simulink library "threeSurfaceThreeTether_cl"  (R2018b)
settings: Solver=VariableStepAuto  StartTime=0.0  StopTime=10.0  RelTol=1e-3
libraries: vrlib x4, aeroSurface_ul x4, apparentWind_ul x1, eulAng2RotMat_ul x1, vectorNormalizer_ul x1, sixDoFKinematics_ul x1
settings Model: Creator=mcobb  LastModifiedBy=mcobb

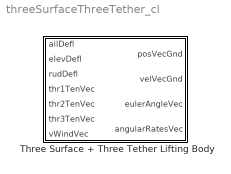
== system threeSurfaceThreeTether_cl ==
  Three Surface + Three Tether Lifting Body : Subsystem  mask{rho=1.225, vol=1, grav=9.81, thr1PosVec=[1 0 0], thr2PosVec=[1 0 0], thr3PosVec=[1 0 0], CB2CMVec=[1 0 0], m=1, inertiaMatrix=eye(3), initPos=[0 0 0], initVel=[0 0 0], initEulerAngles=[0 0 0], initAngRates=[0 0 0], hStabWingAeroCentVec=[0 0 0], hStabRotVec=[1 0 0], hStabChordVec=[0 1 0], hStabRefArea=1, hStabLiftCoeffFitParams=[1 0], hStabDragCoeffFitParams=[1 0 0], vStabWingAeroCentVec=[0 0 0], vStabRotVec=[1 0 0], vStabChordVec=[0 1 0], vStabRefArea=1, vStabLiftCoeffFitParams=[1 0], vStabDragCoeffFitParams=[1 0 0], prtWingAeroCentVec=[0 0 0], prtRotVec=[1 0 0], prtChordVec=[0 1 0], prtRefArea=1, prtLiftCoeffFitParams=[1 0], prtDragCoeffFitParams=[1 0 0], sbdWingAeroCentVec=[0 0 0], sbdRotVec=[1 0 0], sbdChordVec=[0 1 0], sbdRefArea=1, sbdLiftCoeffFitParams=[1 0], sbdDragCoeffFitParams=[1 0 0]}
      mask prompts: rho "Fuild Density"; vol "Volume"; grav "Gravity"; thr1PosVec "Tether 1"; thr2PosVec "Tether 2"; thr3PosVec "Tether 3"; CB2CMVec "CoM 2 CoB Vec"; m "Mass"; inertiaMatrix "Inertia matrix"; initPos "Initial position vec"; initVel "Initial velocity vec"; initEulerAngles "Initial euler angles"; initAngRates "Initial angular rates vec"; hStabWingAeroCentVec "Aerodynamic Center Vec"; hStabRotVec "Spanwise Rotation Vector"; hStabChordVec "Chord Direction Vec"; hStabRefArea "Ref Area"; hStabLiftCoeffFitParams "Lift Coefficient Fit Parameters"; hStabDragCoeffFitParams "Drag Coefficient Fit Parameters"; vStabWingAeroCentVec "Aerodynamic Center Vec"; vStabRotVec "Spanwise Rotation Vector"; vStabChordVec "Chord Direction Vec"; vStabRefArea "Ref Area"; vStabLiftCoeffFitParams "Lift Coefficient Fit Parameters"; vStabDragCoeffFitParams "Drag Coefficient Fit Parameters"; prtWingAeroCentVec "Aerodynamic Center Vec"; prtRotVec "Spanwise Rotation Vector"; prtChordVec "Chord Direction Vec"; prtRefArea "Ref Area"; prtLiftCoeffFitParams "Lift Coefficient Fit Parameters"; prtDragCoeffFitParams "Drag Coefficient Fit Parameters"; sbdWingAeroCentVec "Aerodynamic Center Vec"; sbdRotVec "Spanwise Rotation Vector"; sbdChordVec "Chord Direction Vec"; sbdRefArea "Ref Area"; sbdLiftCoeffFitParams "Lift Coefficient Fit Parameters"; sbdDragCoeffFitParams "Drag Coefficient Fit Parameters"
      mask DialogControl Container8 Prompt: Parameters
      mask DialogControl ParameterGroupVar Prompt: Environmental
      mask DialogControl Container3 Prompt: Tether attachment positiong vecs in body frame
      mask DialogControl Container4 Prompt: Cent of mass 2 cent of buoy vec
      mask DialogControl Container5 Prompt: Inertial Settings
      mask DialogControl Container11 Prompt: Horz. Stab.
      mask DialogControl Container14 Prompt: Aerodynamic Parameters
      mask DialogControl Container16 Prompt: Vert. Stab.
      mask DialogControl Container15 Prompt: Aerodynamic Parameters
      mask DialogControl Container17 Prompt: Port Wing
      mask DialogControl Container12 Prompt: Aerodynamic Parameters
      mask DialogControl Container18 Prompt: Stb. Wing
      mask DialogControl Container13 Prompt: Aerodynamic Parameters

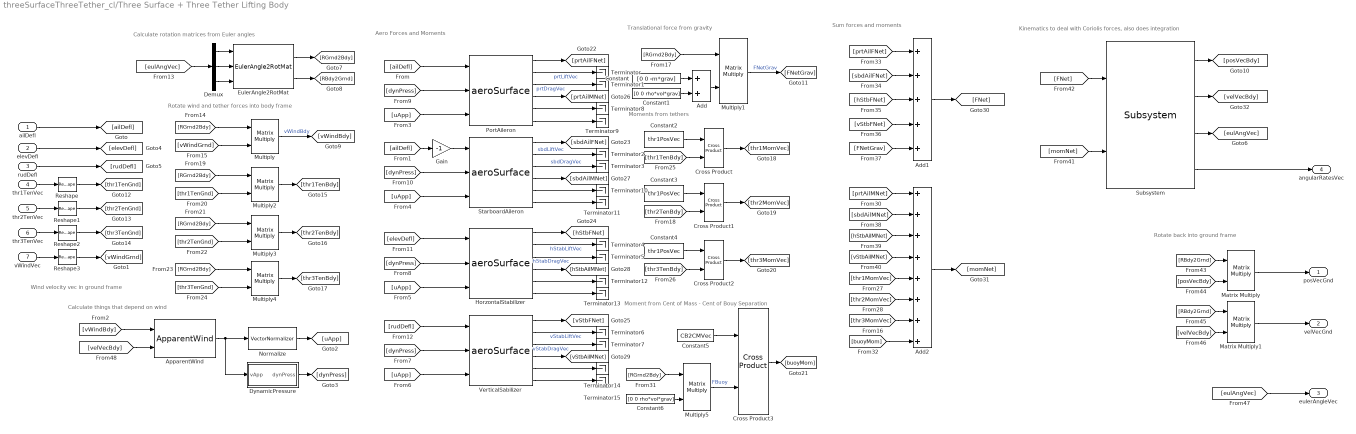
== system threeSurfaceThreeTether_cl/Three Surface + Three Tether Lifting Body ==
  note: Rotate back into ground frame
  note: Kinematics to deal with Coriolis forces, also does integration
  note: Sum forces and moments
  note: Calculate things that depend on wind
  note: Rotate wind and tether forces into body frame
  note: Calculate rotation matrices from Euler angles
  note: Moment from Cent of Mass - Cent of Bouy Separation
  note: Translational force from gravity
  note: Moments from tethers
  note: Aero Forces and Moments
  note: Wind velocity vec in ground frame
  ailDefl : Inport
  elevDefl : Inport  Port=2
  rudDefl : Inport  Port=3
  thr1TenVec : Inport  Port=4
  thr2TenVec : Inport  Port=5
  thr3TenVec : Inport  Port=6
  vWindVec : Inport  Port=7
  Add : Sum
  Add1 : Sum  Inputs=5
  Add2 : Sum  Inputs=++++++++
  ApparentWind : apparentWind_ul/ApparentWind  SystemSampleTime=-1
  Constant : Constant  Value=[0 0 -m*grav]
  Constant1 : Constant  Value=[0 0 rho*vol*grav]
  Constant2 : Constant  Value=thr1PosVec
  Constant3 : Constant  Value=thr1PosVec
  Constant4 : Constant  Value=thr1PosVec
  Constant5 : Constant  Value=CB2CMVec
  Constant6 : Constant  Value=[0 0 rho*vol*grav]
  Cross Product{,1..3} (4 alike) : vrlib/Utilities/Cross Product
      settings: SourceProductBaseCode=VR
  Demux : Demux  Outputs=3
  DynamicPressure : Subsystem  mask{rho=rho}
      mask prompts: rho "Fluid density"
  EulerAngle2RotMat : eulAng2RotMat_ul/EulerAngle2RotMat  SystemSampleTime=-1
  Gain : Gain  Gain=-1
  HorzontalStabilizer : aeroSurface_ul/aeroSurface  rAeroCent=hStabWingAeroCentVec  uSpan=hStabRotVec  uChord=hStabChordVec  ARef=hStabRefArea  ClFitParams=hStabLiftCoeffFitParams  CdFitParams=hStabDragCoeffFitParams
  Matrix Multiply : Product  Multiplication=Matrix(*)
  Matrix Multiply1 : Product  Multiplication=Matrix(*)
  Multiply{,1..5} (6 alike) : Product  Multiplication=Matrix(*)
  "Normalize " : vectorNormalizer_ul/VectorNormalizer   SystemSampleTime=-1
  PortAileron : aeroSurface_ul/aeroSurface  rAeroCent=prtWingAeroCentVec  uSpan=prtRotVec  uChord=prtChordVec  ARef=prtRefArea  ClFitParams=prtLiftCoeffFitParams  CdFitParams=prtDragCoeffFitParams
  Reshape{,1..3} (4 alike) : Reshape
  StarboardAileron : aeroSurface_ul/aeroSurface  rAeroCent=hStabWingAeroCentVec  uSpan=hStabRotVec  uChord=hStabChordVec  ARef=hStabRefArea  ClFitParams=hStabLiftCoeffFitParams  CdFitParams=hStabDragCoeffFitParams
  Subsystem : sixDoFKinematics_ul/Subsystem  m=m  initPos=initPos  initVel=initVel  J=inertiaMatrix  initEulAngs=initEulerAngles  initAngRates=initAngRates
  Terminator{,1..15} (16 alike) : Terminator
  VerticalSabilizer : aeroSurface_ul/aeroSurface  rAeroCent=vStabWingAeroCentVec  uSpan=vStabRotVec  uChord=vStabChordVec  ARef=vStabRefArea  ClFitParams=vStabLiftCoeffFitParams  CdFitParams=vStabDragCoeffFitParams
  posVecGnd : Outport
  velVecGnd : Outport  Port=2
  eulerAngleVec : Outport  Port=3
  angularRatesVec : Outport  Port=4
  wires:
  ailDefl/1 -> [ailDefl]
  Gain/1 -> StarboardAileron/1
  [ailDefl] -> Gain/1
  [ailDefl] -> PortAileron/1
  vWindVec/1 -> Reshape3/1
  [vWindGrnd] -> Multiply/2
  ApparentWind/1 -> "Normalize "/1, DynamicPressure/1(vApp)
  "Normalize "/1 -> [uApp]
  DynamicPressure/1(dynPress) -> [dynPress]
  [uApp] -> PortAileron/3
  [uApp] -> StarboardAileron/3
  [uApp] -> HorzontalStabilizer/3
  [uApp] -> VerticalSabilizer/3
  [dynPress] -> VerticalSabilizer/2
  [dynPress] -> HorzontalStabilizer/2
  [dynPress] -> StarboardAileron/2
  [dynPress] -> PortAileron/2
  elevDefl/1 -> [elevDefl]
  rudDefl/1 -> [rudDefl]
  [elevDefl] -> HorzontalStabilizer/1
  [rudDefl] -> VerticalSabilizer/1
  [eulAngVec] -> Demux/1
  Demux/2 -> EulerAngle2RotMat/2
  Demux/1 -> EulerAngle2RotMat/1
  Demux/3 -> EulerAngle2RotMat/3
  EulerAngle2RotMat/1 -> [RGrnd2Bdy]
  EulerAngle2RotMat/2 -> [RBdy2Grnd]
  [RGrnd2Bdy] -> Multiply/1
  Multiply/1 -> [vWindBdy]  "vWindBdy"
  [vWindBdy] -> ApparentWind/1
  [velVecBdy] -> ApparentWind/2
  [RGrnd2Bdy] -> Multiply1/1
  Constant/1 -> Add/1
  Multiply1/1 -> [FNetGrav]  "FNetGrav"
  Constant1/1 -> Add/2
  Add/1 -> Multiply1/2
  thr1TenVec/1 -> Reshape/1
  thr2TenVec/1 -> Reshape1/1
  thr3TenVec/1 -> Reshape2/1
  Multiply2/1 -> [thr1TenBdy]
  [RGrnd2Bdy] -> Multiply2/1
  [thr1TenGnd] -> Multiply2/2
  [thr2TenGnd] -> Multiply3/2
  [RGrnd2Bdy] -> Multiply3/1
  Multiply3/1 -> [thr2TenBdy]
  Multiply4/1 -> [thr3TenBdy]
  [RGrnd2Bdy] -> Multiply4/1
  [thr3TenGnd] -> Multiply4/2
  [thr1TenBdy] -> Cross Product/2
  Constant2/1 -> Cross Product/1
  Cross Product/1 -> [thr1MomVec]
  Cross Product1/1 -> [thr2MomVec]
  Constant3/1 -> Cross Product1/1
  [thr2TenBdy] -> Cross Product1/2
  [thr3TenBdy] -> Cross Product2/2
  Constant4/1 -> Cross Product2/1
  Cross Product2/1 -> [thr3MomVec]
  Constant6/1 -> Multiply5/2
  Multiply5/1 -> Cross Product3/2  "FBuoy"
  [RGrnd2Bdy] -> Multiply5/1
  Cross Product3/1 -> [buoyMom]
  Constant5/1 -> Cross Product3/1
  PortAileron/1 -> [prtAilFNet]
  StarboardAileron/1 -> [sbdAilFNet]
  HorzontalStabilizer/1 -> [hStbFNet]
  VerticalSabilizer/1 -> [vStbFNet]
  PortAileron/2 -> Terminator/1  "prtLiftVec"
  PortAileron/3 -> Terminator1/1  "prtDragVec"
  StarboardAileron/3 -> Terminator3/1  "sbdDragVec"
  StarboardAileron/2 -> Terminator2/1  "sbdLiftVec"
  HorzontalStabilizer/2 -> Terminator4/1  "hStabLiftVec"
  HorzontalStabilizer/3 -> Terminator5/1  "hStabDragVec"
  VerticalSabilizer/2 -> Terminator6/1  "vStabLiftVec"
  VerticalSabilizer/3 -> Terminator7/1  "vStabDragVec"
  PortAileron/5 -> Terminator8/1
  PortAileron/6 -> Terminator9/1
  StarboardAileron/6 -> Terminator11/1
  StarboardAileron/5 -> Terminator10/1
  HorzontalStabilizer/6 -> Terminator13/1
  HorzontalStabilizer/5 -> Terminator12/1
  VerticalSabilizer/5 -> Terminator14/1
  VerticalSabilizer/6 -> Terminator15/1
  PortAileron/4 -> [prtAilMNet]
  StarboardAileron/4 -> [sbdAilMNet]
  HorzontalStabilizer/4 -> [hStbAilMNet]
  VerticalSabilizer/4 -> [vStbAilMNet]
  [prtAilFNet] -> Add1/1
  [sbdAilFNet] -> Add1/2
  [hStbFNet] -> Add1/3
  [vStbFNet] -> Add1/4
  [FNetGrav] -> Add1/5
  Add1/1 -> [FNet]
  [prtAilMNet] -> Add2/1
  [sbdAilMNet] -> Add2/2
  [hStbAilMNet] -> Add2/3
  [buoyMom] -> Add2/8
  [thr3MomVec] -> Add2/7
  [thr2MomVec] -> Add2/6
  [thr1MomVec] -> Add2/5
  [vStbAilMNet] -> Add2/4
  Add2/1 -> [momNet]
  [momNet] -> Subsystem/2
  [FNet] -> Subsystem/1
  Subsystem/3 -> [eulAngVec]
  Subsystem/1 -> [posVecBdy]
  Subsystem/2 -> [velVecBdy]
  Subsystem/4 -> angularRatesVec/1
  [RBdy2Grnd] -> Matrix Multiply/1
  Matrix Multiply/1 -> posVecGnd/1
  [posVecBdy] -> Matrix Multiply/2
  [velVecBdy] -> Matrix Multiply1/2
  [RBdy2Grnd] -> Matrix Multiply1/1
  Matrix Multiply1/1 -> velVecGnd/1
  [eulAngVec] -> eulerAngleVec/1
  Reshape/1 -> [thr1TenGnd]
  Reshape1/1 -> [thr2TenGnd]
  Reshape2/1 -> [thr3TenGnd]
  Reshape3/1 -> [vWindGrnd]

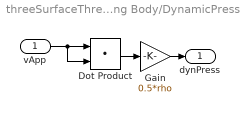
== system threeSurfaceThreeTether_cl/Three Surface + Three Tether Lifting Body/DynamicPressure ==
  vApp : Inport
  Dot Product : DotProduct  InputSameDT=on  OutDataTypeStr=Inherit: Inherit via internal rule
  Gain : Gain  Gain=0.5*rho
  dynPress : Outport
  wires:
  Dot Product/1 -> Gain/1
  vApp/1 -> Dot Product/1, Dot Product/2
  Gain/1 -> dynPress/1
